simulink model "Vehicle_system_Nonlinear_MPC"  (R2024b)
settings: configuration reference "vehicle_nl_system_config" (kept outside this file)
undefined symbols (not defined in the file or in its folder): nl_ref_signal_MAT, path_Tf, plant_ts, TimeStep, u0, x0
settings Model: DataDictionary=sim_data_vehicle_nl.sldd  Creator=tshintai  LastModifiedBy=tshintai
settings ConfigSetRef: SourceName=vehicle_nl_system_config

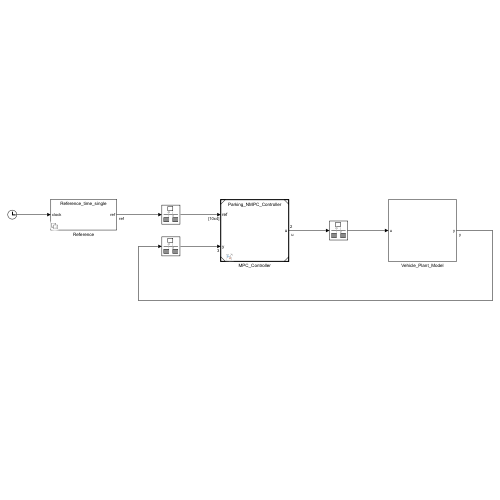
[thumbnail: Simulink's stored preview of the top-level diagram]
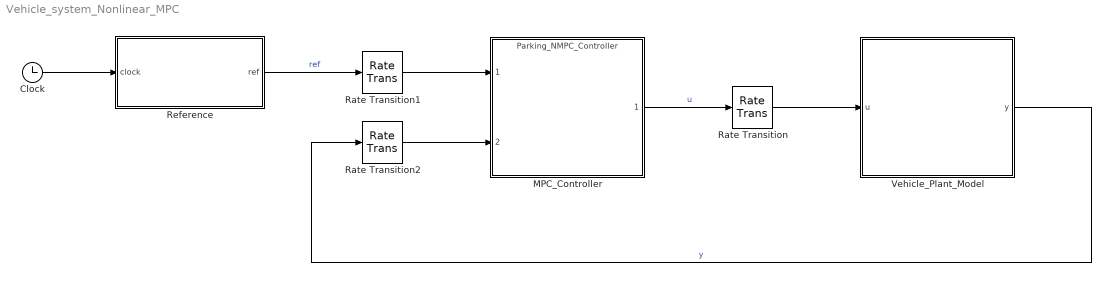
== system Vehicle_system_Nonlinear_MPC ==
  Clock : Clock
  MPC_Controller : ModelReference  ModelNameDialog=Parking_NMPC_Controller  SimulationMode=Normal  ModelReferenceVersion=9.0
  Rate Transition : RateTransition
  Rate Transition1 : RateTransition  OutPortSampleTime=TimeStep
  Rate Transition2 : RateTransition  OutPortSampleTime=TimeStep
  Reference : Subsystem  Variant=on  VariantControl=Choice
  Vehicle_Plant_Model : Subsystem
  wires:
  Rate Transition2/1 -> MPC_Controller/2
  MPC_Controller/1 -> Rate Transition/1  "u"
  Rate Transition/1 -> Vehicle_Plant_Model/1(u)
  Vehicle_Plant_Model/1(y) -> Rate Transition2/1  "y"
  Rate Transition1/1 -> MPC_Controller/1
  Clock/1 -> Reference/1(clock)
  Reference/1(ref) -> Rate Transition1/1  "ref"

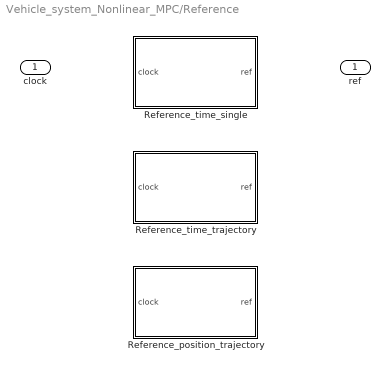
== system Vehicle_system_Nonlinear_MPC/Reference ==
  clock : Inport
  Reference_position_trajectory : Subsystem
  Reference_time_single : Subsystem  VariantControl=ref_VALIANT_TS
  Reference_time_trajectory : Subsystem  VariantControl=ref_VALIANT_TT
  ref : Outport

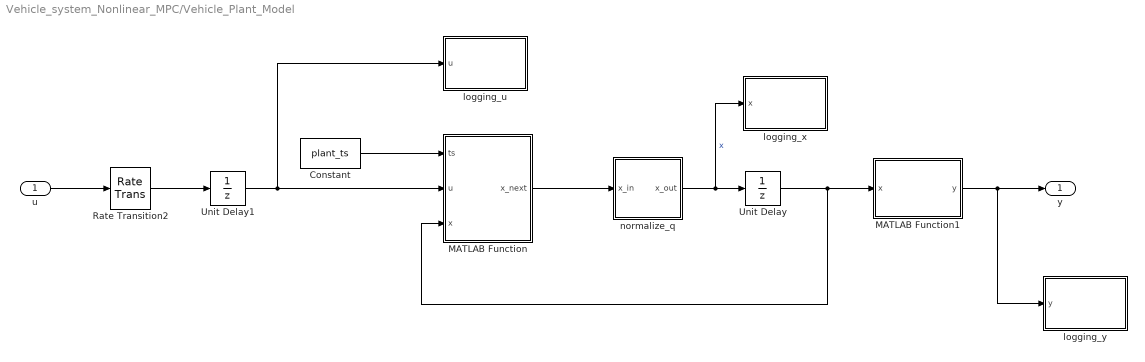
== system Vehicle_system_Nonlinear_MPC/Vehicle_Plant_Model ==
  u : Inport
  Constant : Constant  Value=plant_ts
  MATLAB Function : MATLAB Function  TreatAsAtomicUnit=on
  MATLAB Function1 : MATLAB Function  TreatAsAtomicUnit=on
  Rate Transition2 : RateTransition  OutPortSampleTime=plant_ts
  Unit Delay : UnitDelay  InitialCondition=x0  SampleTime=-1  HasFrameUpgradeWarning=on
  Unit Delay1 : UnitDelay  InitialCondition=u0  SampleTime=-1  HasFrameUpgradeWarning=on
  logging_u : Subsystem
  logging_x : Subsystem
  logging_y : Subsystem
  normalize_q : Subsystem
  y : Outport
  wires:
  Constant/1 -> MATLAB Function/1(ts)
  MATLAB Function/1(x_next) -> normalize_q/1(x_in)
  u/1 -> Rate Transition2/1
  normalize_q/1(x_out) -> logging_x/1(x), Unit Delay/1  "x"
  MATLAB Function1/1(y) -> logging_y/1(y), y/1
  Unit Delay/1 -> MATLAB Function/3(x), MATLAB Function1/1(x)
  Rate Transition2/1 -> Unit Delay1/1
  Unit Delay1/1 -> logging_u/1(u), MATLAB Function/2(u)

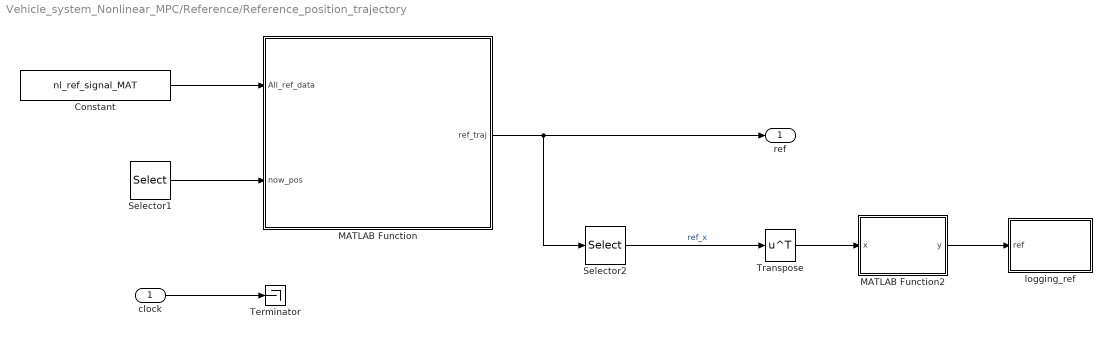
== system Vehicle_system_Nonlinear_MPC/Reference/Reference_position_trajectory ==
  clock : Inport
  Constant : Constant  Value=nl_ref_signal_MAT  VectorParams1D=off
  MATLAB Function : MATLAB Function  TreatAsAtomicUnit=on
  MATLAB Function2 : MATLAB Function  TreatAsAtomicUnit=on
  Selector1 : Selector  InputPortWidth=3  IndexOptions=Index vector (dialog)  Indices=[1 2]  OutputSizes=1
  Selector2 : Selector  NumberOfDimensions=2  InputPortWidth=3  IndexOptions=Index vector (dialog),Select all  Indices=[1],1  OutputSizes=1,1
  Terminator : Terminator
  Transpose : Math  Operator=transpose
  logging_ref : Subsystem
  ref : Outport
  wires:
  Constant/1 -> MATLAB Function/1(All_ref_data)
  Transpose/1 -> MATLAB Function2/1(x)
  MATLAB Function/1(ref_traj) -> ref/1, Selector2/1
  Selector1/1 -> MATLAB Function/2(now_pos)
  clock/1 -> Terminator/1
  Selector2/1 -> Transpose/1  "ref_x"
  MATLAB Function2/1(y) -> logging_ref/1(ref)

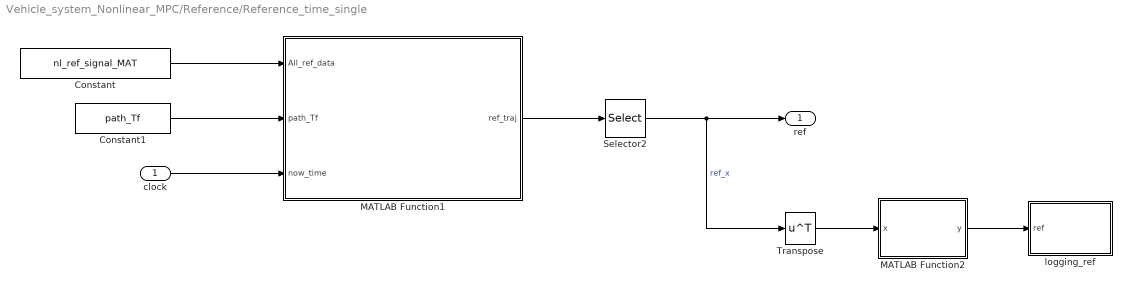
== system Vehicle_system_Nonlinear_MPC/Reference/Reference_time_single ==
  clock : Inport
  Constant : Constant  Value=nl_ref_signal_MAT  VectorParams1D=off
  Constant1 : Constant  Value=path_Tf
  MATLAB Function1 : MATLAB Function  TreatAsAtomicUnit=on
  MATLAB Function2 : MATLAB Function  TreatAsAtomicUnit=on
  Selector2 : Selector  NumberOfDimensions=2  InputPortWidth=3  IndexOptions=Index vector (dialog),Select all  Indices=[1],1  OutputSizes=1,1
  Transpose : Math  Operator=transpose
  logging_ref : Subsystem
  ref : Outport
  wires:
  Constant/1 -> MATLAB Function1/1(All_ref_data)
  Transpose/1 -> MATLAB Function2/1(x)
  MATLAB Function1/1(ref_traj) -> Selector2/1
  Constant1/1 -> MATLAB Function1/2(path_Tf)
  clock/1 -> MATLAB Function1/3(now_time)
  Selector2/1 -> Transpose/1, ref/1  "ref_x"
  MATLAB Function2/1(y) -> logging_ref/1(ref)

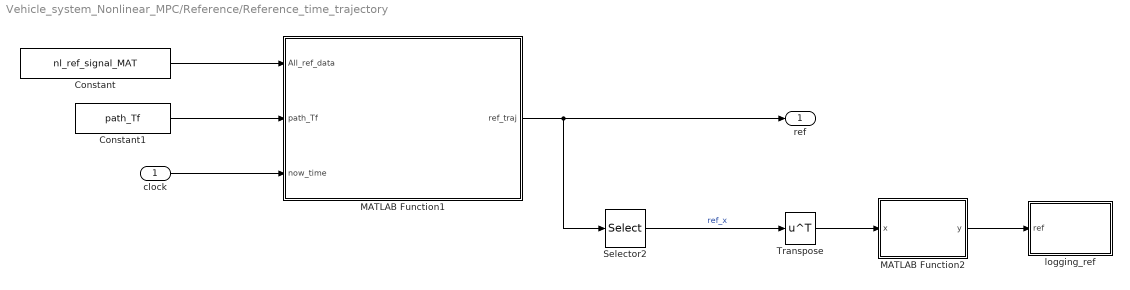
== system Vehicle_system_Nonlinear_MPC/Reference/Reference_time_trajectory ==
  clock : Inport
  Constant : Constant  Value=nl_ref_signal_MAT  VectorParams1D=off
  Constant1 : Constant  Value=path_Tf
  MATLAB Function1 : MATLAB Function  TreatAsAtomicUnit=on
  MATLAB Function2 : MATLAB Function  TreatAsAtomicUnit=on
  Selector2 : Selector  NumberOfDimensions=2  InputPortWidth=3  IndexOptions=Index vector (dialog),Select all  Indices=[1],1  OutputSizes=1,1
  Transpose : Math  Operator=transpose
  logging_ref : Subsystem
  ref : Outport
  wires:
  MATLAB Function2/1(y) -> logging_ref/1(ref)
  Selector2/1 -> Transpose/1  "ref_x"
  clock/1 -> MATLAB Function1/3(now_time)
  Constant1/1 -> MATLAB Function1/2(path_Tf)
  MATLAB Function1/1(ref_traj) -> Selector2/1, ref/1
  Transpose/1 -> MATLAB Function2/1(x)
  Constant/1 -> MATLAB Function1/1(All_ref_data)

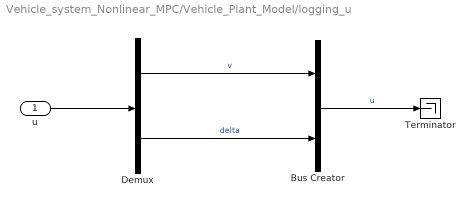
== system Vehicle_system_Nonlinear_MPC/Vehicle_Plant_Model/logging_u ==
  u : Inport
  Bus Creator : BusCreator  Inputs=2
  Demux : Demux  Outputs=2
  Terminator : Terminator
  wires:
  Bus Creator/1 -> Terminator/1  "u"
  Demux/2 -> Bus Creator/2  "delta"
  u/1 -> Demux/1
  Demux/1 -> Bus Creator/1  "v"

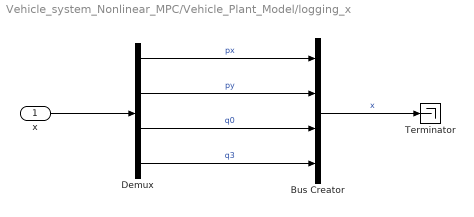
== system Vehicle_system_Nonlinear_MPC/Vehicle_Plant_Model/logging_x ==
  x : Inport
  Bus Creator : BusCreator  Inputs=4
  Demux : Demux
  Terminator : Terminator
  wires:
  Demux/1 -> Bus Creator/1  "px"
  x/1 -> Demux/1
  Demux/2 -> Bus Creator/2  "py"
  Bus Creator/1 -> Terminator/1  "x"
  Demux/3 -> Bus Creator/3  "q0"
  Demux/4 -> Bus Creator/4  "q3"

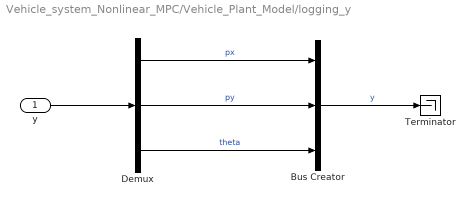
== system Vehicle_system_Nonlinear_MPC/Vehicle_Plant_Model/logging_y ==
  y : Inport
  Bus Creator : BusCreator  Inputs=3
  Demux : Demux  Outputs=3
  Terminator : Terminator
  wires:
  Demux/3 -> Bus Creator/3  "theta"
  Bus Creator/1 -> Terminator/1  "y"
  Demux/2 -> Bus Creator/2  "py"
  y/1 -> Demux/1
  Demux/1 -> Bus Creator/1  "px"

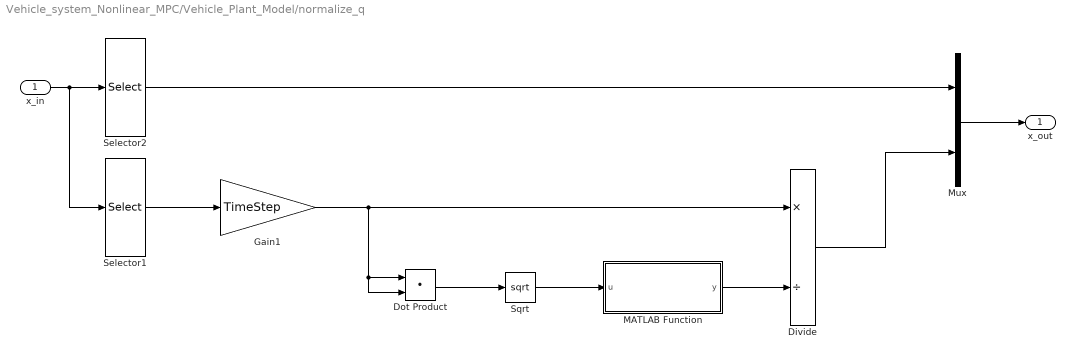
== system Vehicle_system_Nonlinear_MPC/Vehicle_Plant_Model/normalize_q ==
  x_in : Inport
  Divide : Product  Inputs=*/
  Dot Product : DotProduct  OutDataTypeStr=Inherit: Inherit via internal rule
  Gain1 : Gain  Gain=TimeStep
  MATLAB Function : MATLAB Function  TreatAsAtomicUnit=on
  Mux : Mux  Inputs=2
  Selector1 : Selector  InputPortWidth=4  IndexOptions=Index vector (dialog)  Indices=[3 4]  OutputSizes=1
  Selector2 : Selector  InputPortWidth=4  IndexOptions=Index vector (dialog)  Indices=[1 2]  OutputSizes=1
  Sqrt : Sqrt
  x_out : Outport
  wires:
  Selector1/1 -> Gain1/1
  Selector2/1 -> Mux/1
  x_in/1 -> Selector2/1, Selector1/1
  MATLAB Function/1(y) -> Divide/2
  Mux/1 -> x_out/1
  Sqrt/1 -> MATLAB Function/1(u)
  Dot Product/1 -> Sqrt/1
  Gain1/1 -> Divide/1, Dot Product/1, Dot Product/2
  Divide/1 -> Mux/2

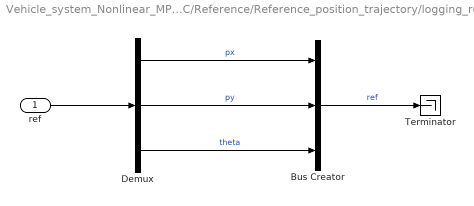
== system Vehicle_system_Nonlinear_MPC/Reference/Reference_position_trajectory/logging_ref ==
  ref : Inport
  Bus Creator : BusCreator  Inputs=3
  Demux : Demux  Outputs=3
  Terminator : Terminator
  wires:
  Demux/3 -> Bus Creator/3  "theta"
  Bus Creator/1 -> Terminator/1  "ref"
  Demux/2 -> Bus Creator/2  "py"
  ref/1 -> Demux/1
  Demux/1 -> Bus Creator/1  "px"

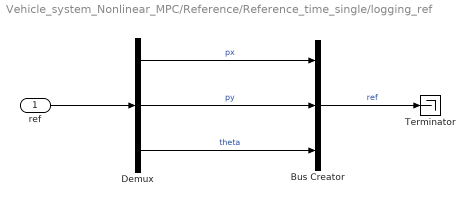
== system Vehicle_system_Nonlinear_MPC/Reference/Reference_time_single/logging_ref ==
  ref : Inport
  Bus Creator : BusCreator  Inputs=3
  Demux : Demux  Outputs=3
  Terminator : Terminator
  wires:
  Demux/3 -> Bus Creator/3  "theta"
  Bus Creator/1 -> Terminator/1  "ref"
  Demux/2 -> Bus Creator/2  "py"
  ref/1 -> Demux/1
  Demux/1 -> Bus Creator/1  "px"

== system Vehicle_system_Nonlinear_MPC/Reference/Reference_time_trajectory/logging_ref ==
  ref : Inport
  Bus Creator : BusCreator  Inputs=3
  Demux : Demux  Outputs=3
  Terminator : Terminator
  wires:
  Demux/1 -> Bus Creator/1  "px"
  ref/1 -> Demux/1
  Demux/2 -> Bus Creator/2  "py"
  Bus Creator/1 -> Terminator/1  "ref"
  Demux/3 -> Bus Creator/3  "theta"

== matlab function Vehicle_system_Nonlinear_MPC/Vehicle_Plant_Model/MATLAB Function ==
  data: ts input; u input; x_next output; x input
function x_next = state_fcn(ts, u, x)

% パラメータ
wb = 2.8;

% 変数
v     = u(1);
delta = u(2);
px    = x(1);
py    = x(2);
q0    = x(3);
q3    = x(4);

x_next = calc_nonlinear_f(ts,delta,px,py,q0,q3,v,wb);

end

== matlab function Vehicle_system_Nonlinear_MPC/Vehicle_Plant_Model/MATLAB Function1 ==
  data: x input; y output
function y = output_fcn(x)

px = x(1);
py = x(2);
q0 = x(3);
q3 = x(4);

y = calc_nonlinear_h(px,py,q0,q3);

if (y(3) > pi)
    y(3) = y(3) - 2 * pi;
elseif (y(3) < -pi)
    y(3) = y(3) + 2 * pi;
else
    % Do Nothing
end

end

== matlab function Vehicle_system_Nonlinear_MPC/Reference/Reference_time_single/MATLAB Function1 ==
  data: All_ref_data input; path_Tf input; ref_traj output; now_time input; NLMPC_Hp parameter
function ref_traj = create_reference_trajectory(All_ref_data, path_Tf, ...
    now_time, NLMPC_Hp)
%% 時刻に応じて与える参照軌道を進める
max_id = size(All_ref_data, 1);
path_id = round(max_id * (now_time / path_Tf)) + 1;

%% 見つけた指令値点から予測ホライズン分の指令値を出力する
ref_traj = zeros(NLMPC_Hp, 4);

for i = 1:NLMPC_Hp
    ref_id = path_id + i - 1;
    if (ref_id > max_id)
        ref_traj(i, :) = All_ref_data(max_id, :);
    else
        ref_traj(i, :) = All_ref_data(ref_id, :);
    end
end

end

== matlab function Vehicle_system_Nonlinear_MPC/Reference/Reference_time_single/MATLAB Function2 ==
  data: x input; y output
function y = output_fcn(x)

px = x(1);
py = x(2);
q0 = x(3);
q3 = x(4);

y = calc_nonlinear_h(px,py,q0,q3);

if (y(3) > pi)
    y(3) = y(3) - 2 * pi;
elseif (y(3) < -pi)
    y(3) = y(3) + 2 * pi;
else
    % Do Nothing
end

end

== matlab function Vehicle_system_Nonlinear_MPC/Vehicle_Plant_Model/normalize_q/MATLAB Function ==
  data: u input; y output; div_min_MPC parameter
function y = avoid_zero_divide(u, div_min_MPC)

y = avoid_zero_divide(u, div_min_MPC);

end

== matlab function Vehicle_system_Nonlinear_MPC/Reference/Reference_time_trajectory/MATLAB Function1 ==
  data: All_ref_data input; path_Tf input; ref_traj output; now_time input; NLMPC_Hp parameter
function ref_traj = create_reference_trajectory(All_ref_data, path_Tf, ...
    now_time, NLMPC_Hp)
%% 時刻に応じて与える参照軌道を進める
max_id = size(All_ref_data, 1);
path_id = round(max_id * (now_time / path_Tf)) + 1;

%% 見つけた指令値点から予測ホライズン分の指令値を出力する
ref_traj = zeros(NLMPC_Hp, 4);

for i = 1:NLMPC_Hp
    ref_id = path_id + i - 1;
    if (ref_id > max_id)
        ref_traj(i, :) = All_ref_data(max_id, :);
    else
        ref_traj(i, :) = All_ref_data(ref_id, :);
    end
end

end

== matlab function Vehicle_system_Nonlinear_MPC/Reference/Reference_time_trajectory/MATLAB Function2 ==
  data: x input; y output
function y = output_fcn(x)

px = x(1);
py = x(2);
q0 = x(3);
q3 = x(4);

y = calc_nonlinear_h(px,py,q0,q3);

if (y(3) > pi)
    y(3) = y(3) - 2 * pi;
elseif (y(3) < -pi)
    y(3) = y(3) + 2 * pi;
else
    % Do Nothing
end

end

== matlab function Vehicle_system_Nonlinear_MPC/Reference/Reference_position_trajectory/MATLAB Function ==
  data: All_ref_data input; ref_traj output; now_pos input; NLMPC_Hp parameter
function ref_traj = create_reference_trajectory(All_ref_data, now_pos, NLMPC_Hp)
%% 今の位置から最も近い軌道指令値点を探す
diff_MAT = zeros(size(All_ref_data(:, 1:2)));
for i = 1:size(All_ref_data, 1)
    diff_MAT(i, :) = All_ref_data(i, 1:2) - now_pos';
end
diff_vec = sum(diff_MAT .^ 2, 2);
[~, diff_min_id] = min(diff_vec);

%% 見つけた指令値点から予測ホライズン分の指令値を出力する
ref_traj = zeros(NLMPC_Hp, 4);
max_id = size(All_ref_data, 1);

for i = 1:NLMPC_Hp
    ref_id = diff_min_id + i - 1;
    if (ref_id > max_id)
        ref_traj(i, :) = All_ref_data(max_id, :);
    else
        ref_traj(i, :) = All_ref_data(ref_id, :);
    end
end

end

== matlab function Vehicle_system_Nonlinear_MPC/Reference/Reference_position_trajectory/MATLAB Function2 ==
  data: x input; y output
function y = output_fcn(x)

px = x(1);
py = x(2);
q0 = x(3);
q3 = x(4);

y = calc_nonlinear_h(px,py,q0,q3);

if (y(3) > pi)
    y(3) = y(3) - 2 * pi;
elseif (y(3) < -pi)
    y(3) = y(3) + 2 * pi;
else
    % Do Nothing
end

end
